simulink model "ANNModel"  (R2020a)
(part 3 of 4)

      mask Display: e = 0.06;c1 = [120 150 230]/255;c2 = ([120 150 230]+0)/383;c3 = ([120 150 230]+128)/383;patch([0 1 1 0],[0 0 1 1],c1);patch([0 1 1 1-e 1-e 0+e],[0 0 1 1-e 0+e 0+e],c2);patch([0 0 1 1-e 0+e 0+e],[0 1 1 1-e 1-e 0+e],c3);plot([0 1 1 0 0],[0 0 1 1 0]);disp('Weights');
  "IW{1,1}(65,:)'" : Constant  Value=[2.01048119893450660811140551231801509857177734375;0.70504892799710316975136947803548537194728851318359375;1.0239440787284330713902136267279274761676788330078125;-1.879350995276042990411724531440995633602142333984375;0.073074914998111084596388309364556334912776947021484375;-1.81261331413633097753290712716989219188690185546875]
      mask Display: e = 0.06;c1 = [120 150 230]/255;c2 = ([120 150 230]+0)/383;c3 = ([120 150 230]+128)/383;patch([0 1 1 0],[0 0 1 1],c1);patch([0 1 1 1-e 1-e 0+e],[0 0 1 1-e 0+e 0+e],c2);patch([0 0 1 1-e 0+e 0+e],[0 1 1 1-e 1-e 0+e],c3);plot([0 1 1 0 0],[0 0 1 1 0]);disp('Weights');
  "IW{1,1}(66,:)'" : Constant  Value=[2.0117467473955681356301283813081681728363037109375;-0.99690094486517699667871283963904716074466705322265625;-1.6194830683528735892906524895806796848773956298828125;-0.053959642446421617056895314590292400680482387542724609375;-1.2621517663738981429588648097706027328968048095703125;1.5627971201349948326964067746303044259548187255859375]
      mask Display: e = 0.06;c1 = [120 150 230]/255;c2 = ([120 150 230]+0)/383;c3 = ([120 150 230]+128)/383;patch([0 1 1 0],[0 0 1 1],c1);patch([0 1 1 1-e 1-e 0+e],[0 0 1 1-e 0+e 0+e],c2);patch([0 0 1 1-e 0+e 0+e],[0 1 1 1-e 1-e 0+e],c3);plot([0 1 1 0 0],[0 0 1 1 0]);disp('Weights');
  "IW{1,1}(67,:)'" : Constant  Value=[-0.55468640388907808347340733234887011349201202392578125;-1.8072998120137355737568896074662916362285614013671875;1.4084537325886230529903286878834478557109832763671875;-2.26489197227907990139783578342758119106292724609375;0.6111699850104539422090965672396123409271240234375;0.91598803965291397677361828755238093435764312744140625]
      mask Display: e = 0.06;c1 = [120 150 230]/255;c2 = ([120 150 230]+0)/383;c3 = ([120 150 230]+128)/383;patch([0 1 1 0],[0 0 1 1],c1);patch([0 1 1 1-e 1-e 0+e],[0 0 1 1-e 0+e 0+e],c2);patch([0 0 1 1-e 0+e 0+e],[0 1 1 1-e 1-e 0+e],c3);plot([0 1 1 0 0],[0 0 1 1 0]);disp('Weights');
  "IW{1,1}(68,:)'" : Constant  Value=[-1.80237433028097182585725022363476455211639404296875;-1.3680544505017240286548485528328455984592437744140625;-0.2461647671690337102479162467716378159821033477783203125;2.514594913903392292553462539217434823513031005859375;-0.57581860612485924466596998172462917864322662353515625;-0.78655755851765551955878663648036308586597442626953125]
      mask Display: e = 0.06;c1 = [120 150 230]/255;c2 = ([120 150 230]+0)/383;c3 = ([120 150 230]+128)/383;patch([0 1 1 0],[0 0 1 1],c1);patch([0 1 1 1-e 1-e 0+e],[0 0 1 1-e 0+e 0+e],c2);patch([0 0 1 1-e 0+e 0+e],[0 1 1 1-e 1-e 0+e],c3);plot([0 1 1 0 0],[0 0 1 1 0]);disp('Weights');
  "IW{1,1}(69,:)'" : Constant  Value=[-0.59530258623193754718982972917729057371616363525390625;1.59112786464784594642196680069901049137115478515625;-2.26450311348175947756544701405800879001617431640625;-0.3097487128205684836501632162253372371196746826171875;1.613861410603679047426339820958673954010009765625;1.125806634448195620024080199073068797588348388671875]
      mask Display: e = 0.06;c1 = [120 150 230]/255;c2 = ([120 150 230]+0)/383;c3 = ([120 150 230]+128)/383;patch([0 1 1 0],[0 0 1 1],c1);patch([0 1 1 1-e 1-e 0+e],[0 0 1 1-e 0+e 0+e],c2);patch([0 0 1 1-e 0+e 0+e],[0 1 1 1-e 1-e 0+e],c3);plot([0 1 1 0 0],[0 0 1 1 0]);disp('Weights');
  "IW{1,1}(7,:)'" : Constant  Value=[2.080524884143426067595328277093358337879180908203125;-0.7775232926412154466078163750353269279003143310546875;0.9697298836179928382961179522681050002574920654296875;0.358211071578419082417354957215138711035251617431640625;0.298192303849937168092054662338341586291790008544921875;2.477504528026019503528232235112227499485015869140625]
      mask Display: e = 0.06;c1 = [120 150 230]/255;c2 = ([120 150 230]+0)/383;c3 = ([120 150 230]+128)/383;patch([0 1 1 0],[0 0 1 1],c1);patch([0 1 1 1-e 1-e 0+e],[0 0 1 1-e 0+e 0+e],c2);patch([0 0 1 1-e 0+e 0+e],[0 1 1 1-e 1-e 0+e],c3);plot([0 1 1 0 0],[0 0 1 1 0]);disp('Weights');
  "IW{1,1}(70,:)'" : Constant  Value=[1.6828954502047734909098153366358019411563873291015625;-0.5070254242972465075212085139355622231960296630859375;-0.928092842787103133872506077750585973262786865234375;1.9536372420043848219251003683893941342830657958984375;0.781021096974864992290576992672868072986602783203125;-1.3177014176442802817490473898942582309246063232421875]
      mask Display: e = 0.06;c1 = [120 150 230]/255;c2 = ([120 150 230]+0)/383;c3 = ([120 150 230]+128)/383;patch([0 1 1 0],[0 0 1 1],c1);patch([0 1 1 1-e 1-e 0+e],[0 0 1 1-e 0+e 0+e],c2);patch([0 0 1 1-e 0+e 0+e],[0 1 1 1-e 1-e 0+e],c3);plot([0 1 1 0 0],[0 0 1 1 0]);disp('Weights');
  "IW{1,1}(71,:)'" : Constant  Value=[0.368726779884062716430292994118644855916500091552734375;1.8550446553590498321995028163655661046504974365234375;1.593744001707899204944851589971221983432769775390625;1.76085446830551273222909003379754722118377685546875;-0.8197428602423286747580277733504772186279296875;-1.6958015554827239323998355757794342935085296630859375]
      mask Display: e = 0.06;c1 = [120 150 230]/255;c2 = ([120 150 230]+0)/383;c3 = ([120 150 230]+128)/383;patch([0 1 1 0],[0 0 1 1],c1);patch([0 1 1 1-e 1-e 0+e],[0 0 1 1-e 0+e 0+e],c2);patch([0 0 1 1-e 0+e 0+e],[0 1 1 1-e 1-e 0+e],c3);plot([0 1 1 0 0],[0 0 1 1 0]);disp('Weights');
  "IW{1,1}(72,:)'" : Constant  Value=[0.5679211220119906311509794250014238059520721435546875;-1.9063634182099631342310885884216986596584320068359375;2.080709917020935773024348236504010856151580810546875;0.88571993688351413620551966232596896588802337646484375;1.580666977905989423192067988566122949123382568359375;-0.91547499703120871483719156458391807973384857177734375]
      mask Display: e = 0.06;c1 = [120 150 230]/255;c2 = ([120 150 230]+0)/383;c3 = ([120 150 230]+128)/383;patch([0 1 1 0],[0 0 1 1],c1);patch([0 1 1 1-e 1-e 0+e],[0 0 1 1-e 0+e 0+e],c2);patch([0 0 1 1-e 0+e 0+e],[0 1 1 1-e 1-e 0+e],c3);plot([0 1 1 0 0],[0 0 1 1 0]);disp('Weights');
  "IW{1,1}(73,:)'" : Constant  Value=[1.7013941327240307277435249488917179405689239501953125;-1.711245018954081320572413460467942059040069580078125;-1.9156052438883619526421853151987306773662567138671875;-0.5773401582797867970242577939643524587154388427734375;0.75396007815125443141113237288664095103740692138671875;-1.36309234224011088798533819499425590038299560546875]
      mask Display: e = 0.06;c1 = [120 150 230]/255;c2 = ([120 150 230]+0)/383;c3 = ([120 150 230]+128)/383;patch([0 1 1 0],[0 0 1 1],c1);patch([0 1 1 1-e 1-e 0+e],[0 0 1 1-e 0+e 0+e],c2);patch([0 0 1 1-e 0+e 0+e],[0 1 1 1-e 1-e 0+e],c3);plot([0 1 1 0 0],[0 0 1 1 0]);disp('Weights');
  "IW{1,1}(74,:)'" : Constant  Value=[-0.94192561738903834989145025247125886380672454833984375;0.498722087201574904025136447671684436500072479248046875;1.7897416372002818985009753305348567664623260498046875;0.6078816384620313595377183446544222533702850341796875;1.9722406625421375903073339941329322755336761474609375;1.9486683235501425226487981490208767354488372802734375]
      mask Display: e = 0.06;c1 = [120 150 230]/255;c2 = ([120 150 230]+0)/383;c3 = ([120 150 230]+128)/383;patch([0 1 1 0],[0 0 1 1],c1);patch([0 1 1 1-e 1-e 0+e],[0 0 1 1-e 0+e 0+e],c2);patch([0 0 1 1-e 0+e 0+e],[0 1 1 1-e 1-e 0+e],c3);plot([0 1 1 0 0],[0 0 1 1 0]);disp('Weights');
  "IW{1,1}(75,:)'" : Constant  Value=[-1.260584968979301390135105975787155330181121826171875;-1.583156214564680031031684848130680620670318603515625;2.441439519515121947534908031229861080646514892578125;0.55855832865015775379191609317786060273647308349609375;0.6561667140789542163048508882638998329639434814453125;1.272402122910108346331981010735034942626953125]
      mask Display: e = 0.06;c1 = [120 150 230]/255;c2 = ([120 150 230]+0)/383;c3 = ([120 150 230]+128)/383;patch([0 1 1 0],[0 0 1 1],c1);patch([0 1 1 1-e 1-e 0+e],[0 0 1 1-e 0+e 0+e],c2);patch([0 0 1 1-e 0+e 0+e],[0 1 1 1-e 1-e 0+e],c3);plot([0 1 1 0 0],[0 0 1 1 0]);disp('Weights');
  "IW{1,1}(76,:)'" : Constant  Value=[-1.5620861437300437302155842189677059650421142578125;1.992427053506375056457500249962322413921356201171875;1.258342771929712444745064203743822872638702392578125;1.707625962939272046270389182609505951404571533203125;-1.290657099160629872613981206086464226245880126953125;-0.48084772219861904307691702342708595097064971923828125]
      mask Display: e = 0.06;c1 = [120 150 230]/255;c2 = ([120 150 230]+0)/383;c3 = ([120 150 230]+128)/383;patch([0 1 1 0],[0 0 1 1],c1);patch([0 1 1 1-e 1-e 0+e],[0 0 1 1-e 0+e 0+e],c2);patch([0 0 1 1-e 0+e 0+e],[0 1 1 1-e 1-e 0+e],c3);plot([0 1 1 0 0],[0 0 1 1 0]);disp('Weights');
  "IW{1,1}(77,:)'" : Constant  Value=[2.38897071465850796556651403079740703105926513671875;1.222965272013324611322104829014278948307037353515625;-0.027361505594901559812459623799441033042967319488525390625;0.66122149176862887731687123960000462830066680908203125;-2.06411195961103910434530916973017156124114990234375;-0.64254666059662868260460300007252953946590423583984375]
      mask Display: e = 0.06;c1 = [120 150 230]/255;c2 = ([120 150 230]+0)/383;c3 = ([120 150 230]+128)/383;patch([0 1 1 0],[0 0 1 1],c1);patch([0 1 1 1-e 1-e 0+e],[0 0 1 1-e 0+e 0+e],c2);patch([0 0 1 1-e 0+e 0+e],[0 1 1 1-e 1-e 0+e],c3);plot([0 1 1 0 0],[0 0 1 1 0]);disp('Weights');
  "IW{1,1}(78,:)'" : Constant  Value=[1.5807466651896839859858800991787575185298919677734375;-0.454131662141270542321080938563682138919830322265625;-0.0263047701204904525729144637580247945152223110198974609375;2.028618506100027918392925130319781601428985595703125;2.260376707315643773910096570034511387348175048828125;0.80948892294460350615992183520575053989887237548828125]
      mask Display: e = 0.06;c1 = [120 150 230]/255;c2 = ([120 150 230]+0)/383;c3 = ([120 150 230]+128)/383;patch([0 1 1 0],[0 0 1 1],c1);patch([0 1 1 1-e 1-e 0+e],[0 0 1 1-e 0+e 0+e],c2);patch([0 0 1 1-e 0+e 0+e],[0 1 1 1-e 1-e 0+e],c3);plot([0 1 1 0 0],[0 0 1 1 0]);disp('Weights');
  "IW{1,1}(79,:)'" : Constant  Value=[2.220118208990346619913225367781706154346466064453125;-1.188699232582106191102866432629525661468505859375;-0.4175275418580761677134205456241033971309661865234375;1.4656419773650852800273014509002678096294403076171875;0.7852553249964155934748077925178222358226776123046875;-1.6447089272281403271591671000351198017597198486328125]
      mask Display: e = 0.06;c1 = [120 150 230]/255;c2 = ([120 150 230]+0)/383;c3 = ([120 150 230]+128)/383;patch([0 1 1 0],[0 0 1 1],c1);patch([0 1 1 1-e 1-e 0+e],[0 0 1 1-e 0+e 0+e],c2);patch([0 0 1 1-e 0+e 0+e],[0 1 1 1-e 1-e 0+e],c3);plot([0 1 1 0 0],[0 0 1 1 0]);disp('Weights');
  "IW{1,1}(8,:)'" : Constant  Value=[-1.7935003758022334263699804068892262876033782958984375;0.29843868613701862724241209434694610536098480224609375;-2.522651458369499888334530623978935182094573974609375;1.435333277484897696041343806427903473377227783203125;-0.86624895688063741072681978039327077567577362060546875;1.140949827713136688345230140839703381061553955078125]
      mask Display: e = 0.06;c1 = [120 150 230]/255;c2 = ([120 150 230]+0)/383;c3 = ([120 150 230]+128)/383;patch([0 1 1 0],[0 0 1 1],c1);patch([0 1 1 1-e 1-e 0+e],[0 0 1 1-e 0+e 0+e],c2);patch([0 0 1 1-e 0+e 0+e],[0 1 1 1-e 1-e 0+e],c3);plot([0 1 1 0 0],[0 0 1 1 0]);disp('Weights');
  "IW{1,1}(80,:)'" : Constant  Value=[-1.4660404262855089019268461925094015896320343017578125;0.137391382491148961175753129282384179532527923583984375;-1.618076432337868908462041872553527355194091796875;-0.249786630682213572907102161479997448623180389404296875;1.4133332653059607064705005541327409446239471435546875;-2.3278113428096975923153877374716103076934814453125]
      mask Display: e = 0.06;c1 = [120 150 230]/255;c2 = ([120 150 230]+0)/383;c3 = ([120 150 230]+128)/383;patch([0 1 1 0],[0 0 1 1],c1);patch([0 1 1 1-e 1-e 0+e],[0 0 1 1-e 0+e 0+e],c2);patch([0 0 1 1-e 0+e 0+e],[0 1 1 1-e 1-e 0+e],c3);plot([0 1 1 0 0],[0 0 1 1 0]);disp('Weights');
  "IW{1,1}(81,:)'" : Constant  Value=[1.349760271573780645582019133144058287143707275390625;1.299337938580240159325285276281647384166717529296875;1.685136151532043324863252564682625234127044677734375;-1.4301162995443295056219312755274586379528045654296875;-1.4578541018409743035277870149002410471439361572265625;-1.342130206320733432079350677668116986751556396484375]
      mask Display: e = 0.06;c1 = [120 150 230]/255;c2 = ([120 150 230]+0)/383;c3 = ([120 150 230]+128)/383;patch([0 1 1 0],[0 0 1 1],c1);patch([0 1 1 1-e 1-e 0+e],[0 0 1 1-e 0+e 0+e],c2);patch([0 0 1 1-e 0+e 0+e],[0 1 1 1-e 1-e 0+e],c3);plot([0 1 1 0 0],[0 0 1 1 0]);disp('Weights');
  "IW{1,1}(82,:)'" : Constant  Value=[-1.1564335079841121523003266702289693057537078857421875;1.6045249632431026753920377814210951328277587890625;-0.1707455074784754722738711052443250082433223724365234375;-1.23054925190401487355984500027261674404144287109375;-1.9217510104204489351786833140067756175994873046875;-1.8064422267415043421578957349993288516998291015625]
      mask Display: e = 0.06;c1 = [120 150 230]/255;c2 = ([120 150 230]+0)/383;c3 = ([120 150 230]+128)/383;patch([0 1 1 0],[0 0 1 1],c1);patch([0 1 1 1-e 1-e 0+e],[0 0 1 1-e 0+e 0+e],c2);patch([0 0 1 1-e 0+e 0+e],[0 1 1 1-e 1-e 0+e],c3);plot([0 1 1 0 0],[0 0 1 1 0]);disp('Weights');
  "IW{1,1}(83,:)'" : Constant  Value=[0.5525434798745931797014918629429303109645843505859375;-0.78297641469172940542620153792086057364940643310546875;1.1899814291930226328730668683419935405254364013671875;-1.56034484041616305916022611199878156185150146484375;1.688224448772421393272225031978450715541839599609375;2.090889872315254915946525215986184775829315185546875]
      mask Display: e = 0.06;c1 = [120 150 230]/255;c2 = ([120 150 230]+0)/383;c3 = ([120 150 230]+128)/383;patch([0 1 1 0],[0 0 1 1],c1);patch([0 1 1 1-e 1-e 0+e],[0 0 1 1-e 0+e 0+e],c2);patch([0 0 1 1-e 0+e 0+e],[0 1 1 1-e 1-e 0+e],c3);plot([0 1 1 0 0],[0 0 1 1 0]);disp('Weights');
  "IW{1,1}(84,:)'" : Constant  Value=[-1.0400378251397761619756465734099037945270538330078125;-0.4003656826447008487690482070320285856723785400390625;1.203899181446665078709656881983391940593719482421875;-2.44165832008013605758378616883419454097747802734375;1.189183998237047124035825618193484842777252197265625;-1.4440764289649450358155036155949346721172332763671875]
      mask Display: e = 0.06;c1 = [120 150 230]/255;c2 = ([120 150 230]+0)/383;c3 = ([120 150 230]+128)/383;patch([0 1 1 0],[0 0 1 1],c1);patch([0 1 1 1-e 1-e 0+e],[0 0 1 1-e 0+e 0+e],c2);patch([0 0 1 1-e 0+e 0+e],[0 1 1 1-e 1-e 0+e],c3);plot([0 1 1 0 0],[0 0 1 1 0]);disp('Weights');
  "IW{1,1}(85,:)'" : Constant  Value=[0.8747160618415448229967523730010725557804107666015625;2.18178875645201042487997256102971732616424560546875;0.022300118205279752248149094384643831290304660797119140625;0.97434004624297754215689337797812186181545257568359375;1.504238940271345637000877104583196341991424560546875;-1.7932695286497886133503243399900384247303009033203125]
      mask Display: e = 0.06;c1 = [120 150 230]/255;c2 = ([120 150 230]+0)/383;c3 = ([120 150 230]+128)/383;patch([0 1 1 0],[0 0 1 1],c1);patch([0 1 1 1-e 1-e 0+e],[0 0 1 1-e 0+e 0+e],c2);patch([0 0 1 1-e 0+e 0+e],[0 1 1 1-e 1-e 0+e],c3);plot([0 1 1 0 0],[0 0 1 1 0]);disp('Weights');
  "IW{1,1}(86,:)'" : Constant  Value=[-0.76748015571507754994939887183136306703090667724609375;1.995871217805269548506430510315112769603729248046875;0.56976188188804954837252125798841007053852081298828125;-1.2275931546708422903435575790354050695896148681640625;-1.10565299157878715874403496854938566684722900390625;-2.09647477510129487399126446689479053020477294921875]
      mask Display: e = 0.06;c1 = [120 150 230]/255;c2 = ([120 150 230]+0)/383;c3 = ([120 150 230]+128)/383;patch([0 1 1 0],[0 0 1 1],c1);patch([0 1 1 1-e 1-e 0+e],[0 0 1 1-e 0+e 0+e],c2);patch([0 0 1 1-e 0+e 0+e],[0 1 1 1-e 1-e 0+e],c3);plot([0 1 1 0 0],[0 0 1 1 0]);disp('Weights');
  "IW{1,1}(87,:)'" : Constant  Value=[1.197230437629724253412177858990617096424102783203125;1.40566500181630349430861315340735018253326416015625;-1.3964094268680486976563770440407097339630126953125;1.6154375103227938126337903668172657489776611328125;1.966654791485958231334052470629103481769561767578125;-0.67972162141895819953418822478852234780788421630859375]
      mask Display: e = 0.06;c1 = [120 150 230]/255;c2 = ([120 150 230]+0)/383;c3 = ([120 150 230]+128)/383;patch([0 1 1 0],[0 0 1 1],c1);patch([0 1 1 1-e 1-e 0+e],[0 0 1 1-e 0+e 0+e],c2);patch([0 0 1 1-e 0+e 0+e],[0 1 1 1-e 1-e 0+e],c3);plot([0 1 1 0 0],[0 0 1 1 0]);disp('Weights');
  "IW{1,1}(88,:)'" : Constant  Value=[1.6304516892283522633277925706352107226848602294921875;-1.3736763496656794192318784553208388388156890869140625;0.44483588902984527724271401893929578363895416259765625;1.4739599025731531245497762938612140715122222900390625;1.6313313119908581239059230938437394797801971435546875;1.6536407433241464559614541940391063690185546875]
      mask Display: e = 0.06;c1 = [120 150 230]/255;c2 = ([120 150 230]+0)/383;c3 = ([120 150 230]+128)/383;patch([0 1 1 0],[0 0 1 1],c1);patch([0 1 1 1-e 1-e 0+e],[0 0 1 1-e 0+e 0+e],c2);patch([0 0 1 1-e 0+e 0+e],[0 1 1 1-e 1-e 0+e],c3);plot([0 1 1 0 0],[0 0 1 1 0]);disp('Weights');
  "IW{1,1}(89,:)'" : Constant  Value=[-1.3903949160357667036436168928048573434352874755859375;-1.442486504743560882246811161166988313198089599609375;1.8623139859514112881555547573952935636043548583984375;-1.1095803087887825544299857938312925398349761962890625;1.43304779435402895870765860308893024921417236328125;-1.3051489705465388890814892874914221465587615966796875]
      mask Display: e = 0.06;c1 = [120 150 230]/255;c2 = ([120 150 230]+0)/383;c3 = ([120 150 230]+128)/383;patch([0 1 1 0],[0 0 1 1],c1);patch([0 1 1 1-e 1-e 0+e],[0 0 1 1-e 0+e 0+e],c2);patch([0 0 1 1-e 0+e 0+e],[0 1 1 1-e 1-e 0+e],c3);plot([0 1 1 0 0],[0 0 1 1 0]);disp('Weights');
  "IW{1,1}(9,:)'" : Constant  Value=[1.5375136387763734813205473983543924987316131591796875;-0.8821494713086164285442691834759898483753204345703125;0.3772187719624258139816674884059466421604156494140625;-0.3003880985703091255345498211681842803955078125;0.9323409464259195811308700285735540091991424560546875;-2.904923487793350300734118718537501990795135498046875]
      mask Display: e = 0.06;c1 = [120 150 230]/255;c2 = ([120 150 230]+0)/383;c3 = ([120 150 230]+128)/383;patch([0 1 1 0],[0 0 1 1],c1);patch([0 1 1 1-e 1-e 0+e],[0 0 1 1-e 0+e 0+e],c2);patch([0 0 1 1-e 0+e 0+e],[0 1 1 1-e 1-e 0+e],c3);plot([0 1 1 0 0],[0 0 1 1 0]);disp('Weights');
  "IW{1,1}(90,:)'" : Constant  Value=[1.5184504077913583142134257286670617759227752685546875;-1.3996797926597395189673989079892635345458984375;1.8215039780381097056505268483306281268596649169921875;-0.043271435426668329593535844423968228511512279510498046875;-1.8302755620244168799359840704710222780704498291015625;-1.234322808009141514418161023058928549289703369140625]
      mask Display: e = 0.06;c1 = [120 150 230]/255;c2 = ([120 150 230]+0)/383;c3 = ([120 150 230]+128)/383;patch([0 1 1 0],[0 0 1 1],c1);patch([0 1 1 1-e 1-e 0+e],[0 0 1 1-e 0+e 0+e],c2);patch([0 0 1 1-e 0+e 0+e],[0 1 1 1-e 1-e 0+e],c3);plot([0 1 1 0 0],[0 0 1 1 0]);disp('Weights');
  "IW{1,1}(91,:)'" : Constant  Value=[-1.601188860125779545029445216641761362552642822265625;-0.7150400036620798704944945711758919060230255126953125;1.771849009912118244614021023153327405452728271484375;1.64997282245795506838703659013845026493072509765625;-1.0732178290379315033220564146176911890506744384765625;-0.937917244397757254859016029513441026210784912109375]
      mask Display: e = 0.06;c1 = [120 150 230]/255;c2 = ([120 150 230]+0)/383;c3 = ([120 150 230]+128)/383;patch([0 1 1 0],[0 0 1 1],c1);patch([0 1 1 1-e 1-e 0+e],[0 0 1 1-e 0+e 0+e],c2);patch([0 0 1 1-e 0+e 0+e],[0 1 1 1-e 1-e 0+e],c3);plot([0 1 1 0 0],[0 0 1 1 0]);disp('Weights');
  "IW{1,1}(92,:)'" : Constant  Value=[-1.475283360364904705619437663699500262737274169921875;-1.5409209155953400571803513230406679213047027587890625;-1.542457133456730300480330697610042989253997802734375;0.441111122317575710116699383434024639427661895751953125;1.49234985489886984311169726424850523471832275390625;1.753336142642942352409818340674974024295806884765625]
      mask Display: e = 0.06;c1 = [120 150 230]/255;c2 = ([120 150 230]+0)/383;c3 = ([120 150 230]+128)/383;patch([0 1 1 0],[0 0 1 1],c1);patch([0 1 1 1-e 1-e 0+e],[0 0 1 1-e 0+e 0+e],c2);patch([0 0 1 1-e 0+e 0+e],[0 1 1 1-e 1-e 0+e],c3);plot([0 1 1 0 0],[0 0 1 1 0]);disp('Weights');
  "IW{1,1}(93,:)'" : Constant  Value=[0.5103180354935477058830883834161795675754547119140625;-0.5267356663054927334854937726049683988094329833984375;1.705559418843760166595302507630549371242523193359375;-1.483384305068874642330456481431610882282257080078125;1.754864106663573952715751147479750216007232666015625;1.912835037094272383484394595143385231494903564453125]
      mask Display: e = 0.06;c1 = [120 150 230]/255;c2 = ([120 150 230]+0)/383;c3 = ([120 150 230]+128)/383;patch([0 1 1 0],[0 0 1 1],c1);patch([0 1 1 1-e 1-e 0+e],[0 0 1 1-e 0+e 0+e],c2);patch([0 0 1 1-e 0+e 0+e],[0 1 1 1-e 1-e 0+e],c3);plot([0 1 1 0 0],[0 0 1 1 0]);disp('Weights');
  "IW{1,1}(94,:)'" : Constant  Value=[-0.85008614681639393939605042760376818478107452392578125;0.6482276478110897688367231239681132137775421142578125;-0.09204177031547768061958691987456404604017734527587890625;2.116484656135848130276144729577936232089996337890625;-1.674224804591101900541616487316787242889404296875;2.028592762921127334863058422342874109745025634765625]
      mask Display: e = 0.06;c1 = [120 150 230]/255;c2 = ([120 150 230]+0)/383;c3 = ([120 150 230]+128)/383;patch([0 1 1 0],[0 0 1 1],c1);patch([0 1 1 1-e 1-e 0+e],[0 0 1 1-e 0+e 0+e],c2);patch([0 0 1 1-e 0+e 0+e],[0 1 1 1-e 1-e 0+e],c3);plot([0 1 1 0 0],[0 0 1 1 0]);disp('Weights');
  "IW{1,1}(95,:)'" : Constant  Value=[1.717788889432830590209277943358756601810455322265625;-1.44071149550639621139680457417853176593780517578125;-1.7880166159163055628056326895602978765964508056640625;0.054784756890892911951329580233505112119019031524658203125;-0.64336187644923892303694401562097482383251190185546875;1.8761286513127062303141201482503674924373626708984375]
      mask Display: e = 0.06;c1 = [120 150 230]/255;c2 = ([120 150 230]+0)/383;c3 = ([120 150 230]+128)/383;patch([0 1 1 0],[0 0 1 1],c1);patch([0 1 1 1-e 1-e 0+e],[0 0 1 1-e 0+e 0+e],c2);patch([0 0 1 1-e 0+e 0+e],[0 1 1 1-e 1-e 0+e],c3);plot([0 1 1 0 0],[0 0 1 1 0]);disp('Weights');
  "IW{1,1}(96,:)'" : Constant  Value=[0.73270940371238513222351684817112982273101806640625;1.690221914643324385707501278375275433063507080078125;-1.523689354895557901414804291562177240848541259765625;1.4059075983117048647130786775960586965084075927734375;-1.7595262735324437297634858623496256768703460693359375;-1.0741362507868215114825716227642260491847991943359375]
      mask Display: e = 0.06;c1 = [120 150 230]/255;c2 = ([120 150 230]+0)/383;c3 = ([120 150 230]+128)/383;patch([0 1 1 0],[0 0 1 1],c1);patch([0 1 1 1-e 1-e 0+e],[0 0 1 1-e 0+e 0+e],c2);patch([0 0 1 1-e 0+e 0+e],[0 1 1 1-e 1-e 0+e],c3);plot([0 1 1 0 0],[0 0 1 1 0]);disp('Weights');
  "IW{1,1}(97,:)'" : Constant  Value=[2.373324965581665058067528661922551691532135009765625;-0.388207992923925659933814813484787009656429290771484375;-0.93680785978463687602157961009652353823184967041015625;1.62599971122309572280073552974499762058258056640625;0.5220493012121867337782532558776438236236572265625;-1.43323412746766098990747195784933865070343017578125]
      mask Display: e = 0.06;c1 = [120 150 230]/255;c2 = ([120 150 230]+0)/383;c3 = ([120 150 230]+128)/383;patch([0 1 1 0],[0 0 1 1],c1);patch([0 1 1 1-e 1-e 0+e],[0 0 1 1-e 0+e 0+e],c2);patch([0 0 1 1-e 0+e 0+e],[0 1 1 1-e 1-e 0+e],c3);plot([0 1 1 0 0],[0 0 1 1 0]);disp('Weights');
  "IW{1,1}(98,:)'" : Constant  Value=[-2.534170344764564930528649711050093173980712890625;0.0833205235921054276904129665126674808561801910400390625;-2.144254325850507125750254999729804694652557373046875;0.52169866819620736020368667595903389155864715576171875;-0.44172220425603747617770977740292437374591827392578125;-0.83959749441214637233343864863854832947254180908203125]
      mask Display: e = 0.06;c1 = [120 150 230]/255;c2 = ([120 150 230]+0)/383;c3 = ([120 150 230]+128)/383;patch([0 1 1 0],[0 0 1 1],c1);patch([0 1 1 1-e 1-e 0+e],[0 0 1 1-e 0+e 0+e],c2);patch([0 0 1 1-e 0+e 0+e],[0 1 1 1-e 1-e 0+e],c3);plot([0 1 1 0 0],[0 0 1 1 0]);disp('Weights');
  "IW{1,1}(99,:)'" : Constant  Value=[-1.7527693063373590565134918506373651325702667236328125;-1.8417149998273469879705999119323678314685821533203125;1.0694117303640287008903442256269045174121856689453125;-0.272660812748511893754965740299667231738567352294921875;-1.342658201089122815830023682792671024799346923828125;1.622145819694084334372519151656888425350189208984375]
      mask Display: e = 0.06;c1 = [120 150 230]/255;c2 = ([120 150 230]+0)/383;c3 = ([120 150 230]+128)/383;patch([0 1 1 0],[0 0 1 1],c1);patch([0 1 1 1-e 1-e 0+e],[0 0 1 1-e 0+e 0+e],c2);patch([0 0 1 1-e 0+e 0+e],[0 1 1 1-e 1-e 0+e],c3);plot([0 1 1 0 0],[0 0 1 1 0]);disp('Weights');
  Mux : Mux  Inputs=250
      mask Display: e = 0.06;c1 = [120 150 230]/255;c2 = ([120 150 230]+0)/383;c3 = ([120 150 230]+128)/383;patch([0 1 1 0],[0 0 1 1],c1);patch([0 1 1 1-e 1-e 0+e],[0 0 1 1-e 0+e 0+e],c2);patch([0 0 1 1-e 0+e 0+e],[0 1 1 1-e 1-e 0+e],c3);plot([0 1 1 0 0],[0 0 1 1 0]);disp('Mux');
  dotprod{1..250} (250 alike) : neural/Weight Functions/dotprod
  "iz{1,1}" : Outport
      mask Display: e = 0.06;c1 = [120 230 180]/255;c2 = ([120 230 180]+0)/(256+128);c3 = ([120 230 180]+128)/(256+128);patch([0 1 1 0],[0 0 1 1],c1);patch([0 1 1 1-e 1-e 0+e],[0 0 1 1-e 0+e 0+e],c2);patch([0 0 1 1-e 0+e 0+e],[0 1 1 1-e 1-e 0+e],c3);plot([0 1 1 0 0],[0 0 1 1 0]);
  wires:
  "IW{1,1}(1,:)'"/1 -> dotprod1/1
  "pd{1,1}"/1 -> dotprod1/2, dotprod2/2, dotprod3/2, dotprod4/2, dotprod5/2, dotprod6/2, dotprod7/2, dotprod8/2, dotprod9/2, dotprod10/2, dotprod11/2, dotprod12/2, dotprod13/2, dotprod14/2, dotprod15/2, dotprod16/2, dotprod17/2, dotprod18/2, dotprod19/2, dotprod20/2, dotprod21/2, dotprod22/2, dotprod23/2, dotprod24/2, dotprod25/2, dotprod26/2, dotprod27/2, dotprod28/2, dotprod29/2, dotprod30/2, dotprod31/2, dotprod32/2, dotprod33/2, dotprod34/2, dotprod35/2, dotprod36/2, dotprod37/2, dotprod38/2, dotprod39/2, dotprod40/2, dotprod41/2, dotprod42/2, dotprod43/2, dotprod44/2, dotprod45/2, dotprod46/2, dotprod47/2, dotprod48/2, dotprod49/2, dotprod50/2, dotprod51/2, dotprod52/2, dotprod53/2, dotprod54/2, dotprod55/2, dotprod56/2, dotprod57/2, dotprod58/2, dotprod59/2, dotprod60/2, dotprod61/2, dotprod62/2, dotprod63/2, dotprod64/2, dotprod65/2, dotprod66/2, dotprod67/2, dotprod68/2, dotprod69/2, dotprod70/2, dotprod71/2, dotprod72/2, dotprod73/2, dotprod74/2, dotprod75/2, dotprod76/2, dotprod77/2, dotprod78/2, dotprod79/2, dotprod80/2, dotprod81/2, dotprod82/2, dotprod83/2, dotprod84/2, dotprod85/2, dotprod86/2, dotprod87/2, dotprod88/2, dotprod89/2, dotprod90/2, dotprod91/2, dotprod92/2, dotprod93/2, dotprod94/2, dotprod95/2, dotprod96/2, dotprod97/2, dotprod98/2, dotprod99/2, dotprod100/2, dotprod101/2, dotprod102/2, dotprod103/2, dotprod104/2, dotprod105/2, dotprod106/2, dotprod107/2, dotprod108/2, dotprod109/2, dotprod110/2, dotprod111/2, dotprod112/2, dotprod113/2, dotprod114/2, dotprod115/2, dotprod116/2, dotprod117/2, dotprod118/2, dotprod119/2, dotprod120/2, dotprod121/2, dotprod122/2, dotprod123/2, dotprod124/2, dotprod125/2, dotprod126/2, dotprod127/2, dotprod128/2, dotprod129/2, dotprod130/2, dotprod131/2, dotprod132/2, dotprod133/2, dotprod134/2, dotprod135/2, dotprod136/2, dotprod137/2, dotprod138/2, dotprod139/2, dotprod140/2, dotprod141/2, dotprod142/2, dotprod143/2, dotprod144/2, dotprod145/2, dotprod146/2, dotprod147/2, dotprod148/2, dotprod149/2, dotprod150/2, dotprod151/2, dotprod152/2, dotprod153/2, dotprod154/2, dotprod155/2, dotprod156/2, dotprod157/2, dotprod158/2, dotprod159/2, dotprod160/2, dotprod161/2, dotprod162/2, dotprod163/2, dotprod164/2, dotprod165/2, dotprod166/2, dotprod167/2, dotprod168/2, dotprod169/2, dotprod170/2, dotprod171/2, dotprod172/2, dotprod173/2, dotprod174/2, dotprod175/2, dotprod176/2, dotprod177/2, dotprod178/2, dotprod179/2, dotprod180/2, dotprod181/2, dotprod182/2, dotprod183/2, dotprod184/2, dotprod185/2, dotprod186/2, dotprod187/2, dotprod188/2, dotprod189/2, dotprod190/2, dotprod191/2, dotprod192/2, dotprod193/2, dotprod194/2, dotprod195/2, dotprod196/2, dotprod197/2, dotprod198/2, dotprod199/2, dotprod200/2, dotprod201/2, dotprod202/2, dotprod203/2, dotprod204/2, dotprod205/2, dotprod206/2, dotprod207/2, dotprod208/2, dotprod209/2, dotprod210/2, dotprod211/2, dotprod212/2, dotprod213/2, dotprod214/2, dotprod215/2, dotprod216/2, dotprod217/2, dotprod218/2, dotprod219/2, dotprod220/2, dotprod221/2, dotprod222/2, dotprod223/2, dotprod224/2, dotprod225/2, dotprod226/2, dotprod227/2, dotprod228/2, dotprod229/2, dotprod230/2, dotprod231/2, dotprod232/2, dotprod233/2, dotprod234/2, dotprod235/2, dotprod236/2, dotprod237/2, dotprod238/2, dotprod239/2, dotprod240/2, dotprod241/2, dotprod242/2, dotprod243/2, dotprod244/2, dotprod245/2, dotprod246/2, dotprod247/2, dotprod248/2, dotprod249/2, dotprod250/2
  dotprod1/1 -> Mux/1
  "IW{1,1}(2,:)'"/1 -> dotprod2/1
  dotprod2/1 -> Mux/2
  "IW{1,1}(3,:)'"/1 -> dotprod3/1
  dotprod3/1 -> Mux/3
  "IW{1,1}(4,:)'"/1 -> dotprod4/1
  dotprod4/1 -> Mux/4
  "IW{1,1}(5,:)'"/1 -> dotprod5/1
  dotprod5/1 -> Mux/5
  "IW{1,1}(6,:)'"/1 -> dotprod6/1
  dotprod6/1 -> Mux/6
  "IW{1,1}(7,:)'"/1 -> dotprod7/1
  dotprod7/1 -> Mux/7
  "IW{1,1}(8,:)'"/1 -> dotprod8/1
  dotprod8/1 -> Mux/8
  "IW{1,1}(9,:)'"/1 -> dotprod9/1
  dotprod9/1 -> Mux/9
  "IW{1,1}(10,:)'"/1 -> dotprod10/1
  dotprod10/1 -> Mux/10
  "IW{1,1}(11,:)'"/1 -> dotprod11/1
  dotprod11/1 -> Mux/11
  "IW{1,1}(12,:)'"/1 -> dotprod12/1
  dotprod12/1 -> Mux/12
  "IW{1,1}(13,:)'"/1 -> dotprod13/1
  dotprod13/1 -> Mux/13
  "IW{1,1}(14,:)'"/1 -> dotprod14/1
  dotprod14/1 -> Mux/14
  "IW{1,1}(15,:)'"/1 -> dotprod15/1
  dotprod15/1 -> Mux/15
  "IW{1,1}(16,:)'"/1 -> dotprod16/1
  dotprod16/1 -> Mux/16
  "IW{1,1}(17,:)'"/1 -> dotprod17/1
  dotprod17/1 -> Mux/17
  "IW{1,1}(18,:)'"/1 -> dotprod18/1
  dotprod18/1 -> Mux/18
  "IW{1,1}(19,:)'"/1 -> dotprod19/1
  dotprod19/1 -> Mux/19
  "IW{1,1}(20,:)'"/1 -> dotprod20/1
  dotprod20/1 -> Mux/20
  "IW{1,1}(21,:)'"/1 -> dotprod21/1
  dotprod21/1 -> Mux/21
  "IW{1,1}(22,:)'"/1 -> dotprod22/1
  dotprod22/1 -> Mux/22
  "IW{1,1}(23,:)'"/1 -> dotprod23/1
  dotprod23/1 -> Mux/23
  "IW{1,1}(24,:)'"/1 -> dotprod24/1
  dotprod24/1 -> Mux/24
  "IW{1,1}(25,:)'"/1 -> dotprod25/1
  dotprod25/1 -> Mux/25
  "IW{1,1}(26,:)'"/1 -> dotprod26/1
  dotprod26/1 -> Mux/26
  "IW{1,1}(27,:)'"/1 -> dotprod27/1
  dotprod27/1 -> Mux/27
  "IW{1,1}(28,:)'"/1 -> dotprod28/1
  dotprod28/1 -> Mux/28
  "IW{1,1}(29,:)'"/1 -> dotprod29/1
  dotprod29/1 -> Mux/29
  "IW{1,1}(30,:)'"/1 -> dotprod30/1
  dotprod30/1 -> Mux/30
  "IW{1,1}(31,:)'"/1 -> dotprod31/1
  dotprod31/1 -> Mux/31
  "IW{1,1}(32,:)'"/1 -> dotprod32/1
  dotprod32/1 -> Mux/32
  "IW{1,1}(33,:)'"/1 -> dotprod33/1
  dotprod33/1 -> Mux/33
  "IW{1,1}(34,:)'"/1 -> dotprod34/1
  dotprod34/1 -> Mux/34
  "IW{1,1}(35,:)'"/1 -> dotprod35/1
  dotprod35/1 -> Mux/35
  "IW{1,1}(36,:)'"/1 -> dotprod36/1
  dotprod36/1 -> Mux/36
  "IW{1,1}(37,:)'"/1 -> dotprod37/1
  dotprod37/1 -> Mux/37
  "IW{1,1}(38,:)'"/1 -> dotprod38/1
  dotprod38/1 -> Mux/38
  "IW{1,1}(39,:)'"/1 -> dotprod39/1
  dotprod39/1 -> Mux/39
  "IW{1,1}(40,:)'"/1 -> dotprod40/1
  dotprod40/1 -> Mux/40
  "IW{1,1}(41,:)'"/1 -> dotprod41/1
  dotprod41/1 -> Mux/41
  "IW{1,1}(42,:)'"/1 -> dotprod42/1
  dotprod42/1 -> Mux/42
  "IW{1,1}(43,:)'"/1 -> dotprod43/1
  dotprod43/1 -> Mux/43
  "IW{1,1}(44,:)'"/1 -> dotprod44/1
  dotprod44/1 -> Mux/44
  "IW{1,1}(45,:)'"/1 -> dotprod45/1
  dotprod45/1 -> Mux/45
  "IW{1,1}(46,:)'"/1 -> dotprod46/1
  dotprod46/1 -> Mux/46
  "IW{1,1}(47,:)'"/1 -> dotprod47/1
  dotprod47/1 -> Mux/47
  "IW{1,1}(48,:)'"/1 -> dotprod48/1
  dotprod48/1 -> Mux/48
  "IW{1,1}(49,:)'"/1 -> dotprod49/1
  dotprod49/1 -> Mux/49
  "IW{1,1}(50,:)'"/1 -> dotprod50/1
  dotprod50/1 -> Mux/50
  "IW{1,1}(51,:)'"/1 -> dotprod51/1
  dotprod51/1 -> Mux/51
  "IW{1,1}(52,:)'"/1 -> dotprod52/1
  dotprod52/1 -> Mux/52
  "IW{1,1}(53,:)'"/1 -> dotprod53/1
  dotprod53/1 -> Mux/53
  "IW{1,1}(54,:)'"/1 -> dotprod54/1
  dotprod54/1 -> Mux/54
  "IW{1,1}(55,:)'"/1 -> dotprod55/1
  dotprod55/1 -> Mux/55
  "IW{1,1}(56,:)'"/1 -> dotprod56/1
  dotprod56/1 -> Mux/56
  "IW{1,1}(57,:)'"/1 -> dotprod57/1
  dotprod57/1 -> Mux/57
  "IW{1,1}(58,:)'"/1 -> dotprod58/1
  dotprod58/1 -> Mux/58
  "IW{1,1}(59,:)'"/1 -> dotprod59/1
  dotprod59/1 -> Mux/59
  "IW{1,1}(60,:)'"/1 -> dotprod60/1
  dotprod60/1 -> Mux/60
  "IW{1,1}(61,:)'"/1 -> dotprod61/1
  dotprod61/1 -> Mux/61
  "IW{1,1}(62,:)'"/1 -> dotprod62/1
  dotprod62/1 -> Mux/62
  "IW{1,1}(63,:)'"/1 -> dotprod63/1
  dotprod63/1 -> Mux/63
  "IW{1,1}(64,:)'"/1 -> dotprod64/1
  dotprod64/1 -> Mux/64
  "IW{1,1}(65,:)'"/1 -> dotprod65/1
  dotprod65/1 -> Mux/65
  "IW{1,1}(66,:)'"/1 -> dotprod66/1
  dotprod66/1 -> Mux/66
  "IW{1,1}(67,:)'"/1 -> dotprod67/1
  dotprod67/1 -> Mux/67
  "IW{1,1}(68,:)'"/1 -> dotprod68/1
  dotprod68/1 -> Mux/68
  "IW{1,1}(69,:)'"/1 -> dotprod69/1
  dotprod69/1 -> Mux/69
  "IW{1,1}(70,:)'"/1 -> dotprod70/1
  dotprod70/1 -> Mux/70
  "IW{1,1}(71,:)'"/1 -> dotprod71/1
  dotprod71/1 -> Mux/71
  "IW{1,1}(72,:)'"/1 -> dotprod72/1
  dotprod72/1 -> Mux/72
  "IW{1,1}(73,:)'"/1 -> dotprod73/1
  dotprod73/1 -> Mux/73
  "IW{1,1}(74,:)'"/1 -> dotprod74/1
  dotprod74/1 -> Mux/74
  "IW{1,1}(75,:)'"/1 -> dotprod75/1
  dotprod75/1 -> Mux/75
  "IW{1,1}(76,:)'"/1 -> dotprod76/1
  dotprod76/1 -> Mux/76
  "IW{1,1}(77,:)'"/1 -> dotprod77/1
  dotprod77/1 -> Mux/77
  "IW{1,1}(78,:)'"/1 -> dotprod78/1
  dotprod78/1 -> Mux/78
  "IW{1,1}(79,:)'"/1 -> dotprod79/1
  dotprod79/1 -> Mux/79
  "IW{1,1}(80,:)'"/1 -> dotprod80/1
  dotprod80/1 -> Mux/80
  "IW{1,1}(81,:)'"/1 -> dotprod81/1
  dotprod81/1 -> Mux/81
  "IW{1,1}(82,:)'"/1 -> dotprod82/1
  dotprod82/1 -> Mux/82
  "IW{1,1}(83,:)'"/1 -> dotprod83/1
  dotprod83/1 -> Mux/83
  "IW{1,1}(84,:)'"/1 -> dotprod84/1
  dotprod84/1 -> Mux/84
  "IW{1,1}(85,:)'"/1 -> dotprod85/1
  dotprod85/1 -> Mux/85
  "IW{1,1}(86,:)'"/1 -> dotprod86/1
  dotprod86/1 -> Mux/86
  "IW{1,1}(87,:)'"/1 -> dotprod87/1
  dotprod87/1 -> Mux/87
  "IW{1,1}(88,:)'"/1 -> dotprod88/1
  dotprod88/1 -> Mux/88
  "IW{1,1}(89,:)'"/1 -> dotprod89/1
  dotprod89/1 -> Mux/89
  "IW{1,1}(90,:)'"/1 -> dotprod90/1
  dotprod90/1 -> Mux/90
  "IW{1,1}(91,:)'"/1 -> dotprod91/1
  dotprod91/1 -> Mux/91
  "IW{1,1}(92,:)'"/1 -> dotprod92/1
  dotprod92/1 -> Mux/92
  "IW{1,1}(93,:)'"/1 -> dotprod93/1
  dotprod93/1 -> Mux/93
  "IW{1,1}(94,:)'"/1 -> dotprod94/1
  dotprod94/1 -> Mux/94
  "IW{1,1}(95,:)'"/1 -> dotprod95/1
  dotprod95/1 -> Mux/95
  "IW{1,1}(96,:)'"/1 -> dotprod96/1
  dotprod96/1 -> Mux/96
  "IW{1,1}(97,:)'"/1 -> dotprod97/1
  dotprod97/1 -> Mux/97
  "IW{1,1}(98,:)'"/1 -> dotprod98/1
  dotprod98/1 -> Mux/98
  "IW{1,1}(99,:)'"/1 -> dotprod99/1
  dotprod99/1 -> Mux/99
  "IW{1,1}(100,:)'"/1 -> dotprod100/1
  dotprod100/1 -> Mux/100
  "IW{1,1}(101,:)'"/1 -> dotprod101/1
  dotprod101/1 -> Mux/101
  "IW{1,1}(102,:)'"/1 -> dotprod102/1
  dotprod102/1 -> Mux/102
  "IW{1,1}(103,:)'"/1 -> dotprod103/1
  dotprod103/1 -> Mux/103
  "IW{1,1}(104,:)'"/1 -> dotprod104/1
  dotprod104/1 -> Mux/104
  "IW{1,1}(105,:)'"/1 -> dotprod105/1
  dotprod105/1 -> Mux/105
  "IW{1,1}(106,:)'"/1 -> dotprod106/1
  dotprod106/1 -> Mux/106
  "IW{1,1}(107,:)'"/1 -> dotprod107/1
  dotprod107/1 -> Mux/107
  "IW{1,1}(108,:)'"/1 -> dotprod108/1
  dotprod108/1 -> Mux/108
  "IW{1,1}(109,:)'"/1 -> dotprod109/1
  dotprod109/1 -> Mux/109
  "IW{1,1}(110,:)'"/1 -> dotprod110/1
  dotprod110/1 -> Mux/110
  "IW{1,1}(111,:)'"/1 -> dotprod111/1
  dotprod111/1 -> Mux/111
  "IW{1,1}(112,:)'"/1 -> dotprod112/1
  dotprod112/1 -> Mux/112
  "IW{1,1}(113,:)'"/1 -> dotprod113/1
  dotprod113/1 -> Mux/113
  "IW{1,1}(114,:)'"/1 -> dotprod114/1
  dotprod114/1 -> Mux/114
  "IW{1,1}(115,:)'"/1 -> dotprod115/1
  dotprod115/1 -> Mux/115
  "IW{1,1}(116,:)'"/1 -> dotprod116/1
  dotprod116/1 -> Mux/116
  "IW{1,1}(117,:)'"/1 -> dotprod117/1
  dotprod117/1 -> Mux/117
  "IW{1,1}(118,:)'"/1 -> dotprod118/1
  dotprod118/1 -> Mux/118
  "IW{1,1}(119,:)'"/1 -> dotprod119/1
  dotprod119/1 -> Mux/119
  "IW{1,1}(120,:)'"/1 -> dotprod120/1
  dotprod120/1 -> Mux/120
  "IW{1,1}(121,:)'"/1 -> dotprod121/1
  dotprod121/1 -> Mux/121
  "IW{1,1}(122,:)'"/1 -> dotprod122/1
  dotprod122/1 -> Mux/122
  "IW{1,1}(123,:)'"/1 -> dotprod123/1
  dotprod123/1 -> Mux/123
  "IW{1,1}(124,:)'"/1 -> dotprod124/1
  dotprod124/1 -> Mux/124
  "IW{1,1}(125,:)'"/1 -> dotprod125/1
  dotprod125/1 -> Mux/125
  "IW{1,1}(126,:)'"/1 -> dotprod126/1
  dotprod126/1 -> Mux/126
  "IW{1,1}(127,:)'"/1 -> dotprod127/1
  dotprod127/1 -> Mux/127
  "IW{1,1}(128,:)'"/1 -> dotprod128/1
  dotprod128/1 -> Mux/128
  "IW{1,1}(129,:)'"/1 -> dotprod129/1
  dotprod129/1 -> Mux/129
  "IW{1,1}(130,:)'"/1 -> dotprod130/1
  dotprod130/1 -> Mux/130
  "IW{1,1}(131,:)'"/1 -> dotprod131/1
  dotprod131/1 -> Mux/131
  "IW{1,1}(132,:)'"/1 -> dotprod132/1
  dotprod132/1 -> Mux/132
  "IW{1,1}(133,:)'"/1 -> dotprod133/1
  dotprod133/1 -> Mux/133
  "IW{1,1}(134,:)'"/1 -> dotprod134/1
  dotprod134/1 -> Mux/134
  "IW{1,1}(135,:)'"/1 -> dotprod135/1
  dotprod135/1 -> Mux/135
  "IW{1,1}(136,:)'"/1 -> dotprod136/1
  dotprod136/1 -> Mux/136
  "IW{1,1}(137,:)'"/1 -> dotprod137/1
  dotprod137/1 -> Mux/137
  "IW{1,1}(138,:)'"/1 -> dotprod138/1
  dotprod138/1 -> Mux/138
  "IW{1,1}(139,:)'"/1 -> dotprod139/1
  dotprod139/1 -> Mux/139
  "IW{1,1}(140,:)'"/1 -> dotprod140/1
  dotprod140/1 -> Mux/140
  "IW{1,1}(141,:)'"/1 -> dotprod141/1
  dotprod141/1 -> Mux/141
  "IW{1,1}(142,:)'"/1 -> dotprod142/1
  dotprod142/1 -> Mux/142
  "IW{1,1}(143,:)'"/1 -> dotprod143/1
  dotprod143/1 -> Mux/143
  "IW{1,1}(144,:)'"/1 -> dotprod144/1
  dotprod144/1 -> Mux/144
  "IW{1,1}(145,:)'"/1 -> dotprod145/1
  dotprod145/1 -> Mux/145
  "IW{1,1}(146,:)'"/1 -> dotprod146/1
  dotprod146/1 -> Mux/146
  "IW{1,1}(147,:)'"/1 -> dotprod147/1
  dotprod147/1 -> Mux/147
  "IW{1,1}(148,:)'"/1 -> dotprod148/1
  dotprod148/1 -> Mux/148
  "IW{1,1}(149,:)'"/1 -> dotprod149/1
  dotprod149/1 -> Mux/149
  "IW{1,1}(150,:)'"/1 -> dotprod150/1
  dotprod150/1 -> Mux/150
  "IW{1,1}(151,:)'"/1 -> dotprod151/1
  dotprod151/1 -> Mux/151
  "IW{1,1}(152,:)'"/1 -> dotprod152/1
  dotprod152/1 -> Mux/152
  "IW{1,1}(153,:)'"/1 -> dotprod153/1
  dotprod153/1 -> Mux/153
  "IW{1,1}(154,:)'"/1 -> dotprod154/1
  dotprod154/1 -> Mux/154
  "IW{1,1}(155,:)'"/1 -> dotprod155/1
  dotprod155/1 -> Mux/155
  "IW{1,1}(156,:)'"/1 -> dotprod156/1
  dotprod156/1 -> Mux/156
  "IW{1,1}(157,:)'"/1 -> dotprod157/1
  dotprod157/1 -> Mux/157
  "IW{1,1}(158,:)'"/1 -> dotprod158/1
  dotprod158/1 -> Mux/158
  "IW{1,1}(159,:)'"/1 -> dotprod159/1
  dotprod159/1 -> Mux/159
  "IW{1,1}(160,:)'"/1 -> dotprod160/1
  dotprod160/1 -> Mux/160
  "IW{1,1}(161,:)'"/1 -> dotprod161/1
  dotprod161/1 -> Mux/161
  "IW{1,1}(162,:)'"/1 -> dotprod162/1
  dotprod162/1 -> Mux/162
  "IW{1,1}(163,:)'"/1 -> dotprod163/1
  dotprod163/1 -> Mux/163
  "IW{1,1}(164,:)'"/1 -> dotprod164/1
  dotprod164/1 -> Mux/164
  "IW{1,1}(165,:)'"/1 -> dotprod165/1
  dotprod165/1 -> Mux/165
  "IW{1,1}(166,:)'"/1 -> dotprod166/1
  dotprod166/1 -> Mux/166
  "IW{1,1}(167,:)'"/1 -> dotprod167/1
  dotprod167/1 -> Mux/167
  "IW{1,1}(168,:)'"/1 -> dotprod168/1
  dotprod168/1 -> Mux/168
  "IW{1,1}(169,:)'"/1 -> dotprod169/1
  dotprod169/1 -> Mux/169
  "IW{1,1}(170,:)'"/1 -> dotprod170/1
  dotprod170/1 -> Mux/170
  "IW{1,1}(171,:)'"/1 -> dotprod171/1
  dotprod171/1 -> Mux/171
  "IW{1,1}(172,:)'"/1 -> dotprod172/1
  dotprod172/1 -> Mux/172
  "IW{1,1}(173,:)'"/1 -> dotprod173/1
  dotprod173/1 -> Mux/173
  "IW{1,1}(174,:)'"/1 -> dotprod174/1
  dotprod174/1 -> Mux/174
  "IW{1,1}(175,:)'"/1 -> dotprod175/1
  dotprod175/1 -> Mux/175
  "IW{1,1}(176,:)'"/1 -> dotprod176/1
  dotprod176/1 -> Mux/176
  "IW{1,1}(177,:)'"/1 -> dotprod177/1
  dotprod177/1 -> Mux/177
  "IW{1,1}(178,:)'"/1 -> dotprod178/1
  dotprod178/1 -> Mux/178
  "IW{1,1}(179,:)'"/1 -> dotprod179/1
  dotprod179/1 -> Mux/179
  "IW{1,1}(180,:)'"/1 -> dotprod180/1
  dotprod180/1 -> Mux/180
  "IW{1,1}(181,:)'"/1 -> dotprod181/1
  dotprod181/1 -> Mux/181
  "IW{1,1}(182,:)'"/1 -> dotprod182/1
  dotprod182/1 -> Mux/182
  "IW{1,1}(183,:)'"/1 -> dotprod183/1
  dotprod183/1 -> Mux/183
  "IW{1,1}(184,:)'"/1 -> dotprod184/1
  dotprod184/1 -> Mux/184
  "IW{1,1}(185,:)'"/1 -> dotprod185/1
  dotprod185/1 -> Mux/185
  "IW{1,1}(186,:)'"/1 -> dotprod186/1
  dotprod186/1 -> Mux/186
  "IW{1,1}(187,:)'"/1 -> dotprod187/1
  dotprod187/1 -> Mux/187
  "IW{1,1}(188,:)'"/1 -> dotprod188/1
  dotprod188/1 -> Mux/188
  "IW{1,1}(189,:)'"/1 -> dotprod189/1
  dotprod189/1 -> Mux/189
  "IW{1,1}(190,:)'"/1 -> dotprod190/1
  dotprod190/1 -> Mux/190
  "IW{1,1}(191,:)'"/1 -> dotprod191/1
  dotprod191/1 -> Mux/191
  "IW{1,1}(192,:)'"/1 -> dotprod192/1
  dotprod192/1 -> Mux/192
  "IW{1,1}(193,:)'"/1 -> dotprod193/1
  dotprod193/1 -> Mux/193
  "IW{1,1}(194,:)'"/1 -> dotprod194/1
  dotprod194/1 -> Mux/194
  "IW{1,1}(195,:)'"/1 -> dotprod195/1
  dotprod195/1 -> Mux/195
  "IW{1,1}(196,:)'"/1 -> dotprod196/1
  dotprod196/1 -> Mux/196
  "IW{1,1}(197,:)'"/1 -> dotprod197/1
  dotprod197/1 -> Mux/197
  "IW{1,1}(198,:)'"/1 -> dotprod198/1
  dotprod198/1 -> Mux/198
  "IW{1,1}(199,:)'"/1 -> dotprod199/1
  dotprod199/1 -> Mux/199
  "IW{1,1}(200,:)'"/1 -> dotprod200/1
  dotprod200/1 -> Mux/200
  "IW{1,1}(201,:)'"/1 -> dotprod201/1
  dotprod201/1 -> Mux/201
  "IW{1,1}(202,:)'"/1 -> dotprod202/1
  dotprod202/1 -> Mux/202
  "IW{1,1}(203,:)'"/1 -> dotprod203/1
  dotprod203/1 -> Mux/203
  "IW{1,1}(204,:)'"/1 -> dotprod204/1
  dotprod204/1 -> Mux/204
  "IW{1,1}(205,:)'"/1 -> dotprod205/1
  dotprod205/1 -> Mux/205
  "IW{1,1}(206,:)'"/1 -> dotprod206/1
  dotprod206/1 -> Mux/206
  "IW{1,1}(207,:)'"/1 -> dotprod207/1
  dotprod207/1 -> Mux/207
  "IW{1,1}(208,:)'"/1 -> dotprod208/1
  dotprod208/1 -> Mux/208
  "IW{1,1}(209,:)'"/1 -> dotprod209/1
  dotprod209/1 -> Mux/209
  "IW{1,1}(210,:)'"/1 -> dotprod210/1
  dotprod210/1 -> Mux/210
  "IW{1,1}(211,:)'"/1 -> dotprod211/1
  dotprod211/1 -> Mux/211
  "IW{1,1}(212,:)'"/1 -> dotprod212/1
  dotprod212/1 -> Mux/212
  "IW{1,1}(213,:)'"/1 -> dotprod213/1
  dotprod213/1 -> Mux/213
  "IW{1,1}(214,:)'"/1 -> dotprod214/1
  dotprod214/1 -> Mux/214
  "IW{1,1}(215,:)'"/1 -> dotprod215/1
  dotprod215/1 -> Mux/215
  "IW{1,1}(216,:)'"/1 -> dotprod216/1
  dotprod216/1 -> Mux/216
  "IW{1,1}(217,:)'"/1 -> dotprod217/1
  dotprod217/1 -> Mux/217
  "IW{1,1}(218,:)'"/1 -> dotprod218/1
  dotprod218/1 -> Mux/218
  "IW{1,1}(219,:)'"/1 -> dotprod219/1
  dotprod219/1 -> Mux/219
  "IW{1,1}(220,:)'"/1 -> dotprod220/1
  dotprod220/1 -> Mux/220
  "IW{1,1}(221,:)'"/1 -> dotprod221/1
  dotprod221/1 -> Mux/221
  "IW{1,1}(222,:)'"/1 -> dotprod222/1
  dotprod222/1 -> Mux/222
  "IW{1,1}(223,:)'"/1 -> dotprod223/1
  dotprod223/1 -> Mux/223
  "IW{1,1}(224,:)'"/1 -> dotprod224/1
  dotprod224/1 -> Mux/224
  "IW{1,1}(225,:)'"/1 -> dotprod225/1
  dotprod225/1 -> Mux/225
  "IW{1,1}(226,:)'"/1 -> dotprod226/1
  dotprod226/1 -> Mux/226
  "IW{1,1}(227,:)'"/1 -> dotprod227/1
  dotprod227/1 -> Mux/227
  "IW{1,1}(228,:)'"/1 -> dotprod228/1
  dotprod228/1 -> Mux/228
  "IW{1,1}(229,:)'"/1 -> dotprod229/1
  dotprod229/1 -> Mux/229
  "IW{1,1}(230,:)'"/1 -> dotprod230/1
  dotprod230/1 -> Mux/230
  "IW{1,1}(231,:)'"/1 -> dotprod231/1
  dotprod231/1 -> Mux/231
  "IW{1,1}(232,:)'"/1 -> dotprod232/1
  dotprod232/1 -> Mux/232
  "IW{1,1}(233,:)'"/1 -> dotprod233/1
  dotprod233/1 -> Mux/233
  "IW{1,1}(234,:)'"/1 -> dotprod234/1
  dotprod234/1 -> Mux/234
  "IW{1,1}(235,:)'"/1 -> dotprod235/1
  dotprod235/1 -> Mux/235
  "IW{1,1}(236,:)'"/1 -> dotprod236/1
  dotprod236/1 -> Mux/236
  "IW{1,1}(237,:)'"/1 -> dotprod237/1
  dotprod237/1 -> Mux/237
  "IW{1,1}(238,:)'"/1 -> dotprod238/1
  dotprod238/1 -> Mux/238
  "IW{1,1}(239,:)'"/1 -> dotprod239/1
  dotprod239/1 -> Mux/239
  "IW{1,1}(240,:)'"/1 -> dotprod240/1
  dotprod240/1 -> Mux/240
  "IW{1,1}(241,:)'"/1 -> dotprod241/1
  dotprod241/1 -> Mux/241
  "IW{1,1}(242,:)'"/1 -> dotprod242/1
  dotprod242/1 -> Mux/242
  "IW{1,1}(243,:)'"/1 -> dotprod243/1
  dotprod243/1 -> Mux/243
  "IW{1,1}(244,:)'"/1 -> dotprod244/1
  dotprod244/1 -> Mux/244
  "IW{1,1}(245,:)'"/1 -> dotprod245/1
  dotprod245/1 -> Mux/245
  "IW{1,1}(246,:)'"/1 -> dotprod246/1
  dotprod246/1 -> Mux/246
  "IW{1,1}(247,:)'"/1 -> dotprod247/1
  dotprod247/1 -> Mux/247
  "IW{1,1}(248,:)'"/1 -> dotprod248/1
  dotprod248/1 -> Mux/248
  "IW{1,1}(249,:)'"/1 -> dotprod249/1
  dotprod249/1 -> Mux/249
  "IW{1,1}(250,:)'"/1 -> dotprod250/1
  dotprod250/1 -> Mux/250
  Mux/1 -> "iz{1,1}"/1
